simulink library "Autonomous_lib"  (R2023b)
settings: Solver=VariableStepAuto  StartTime=0.0  StopTime=10.0  RelTol=1e-3
undefined symbols (not defined in the file): All_Paths, FloorDistance
libraries: simulink x3
settings Model: Creator=FIRSTMentor  LastModifiedBy=FIRSTMentor

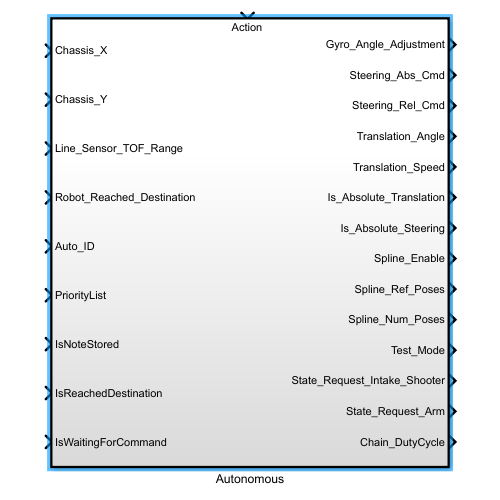
[thumbnail: Simulink's stored preview of the top-level diagram]
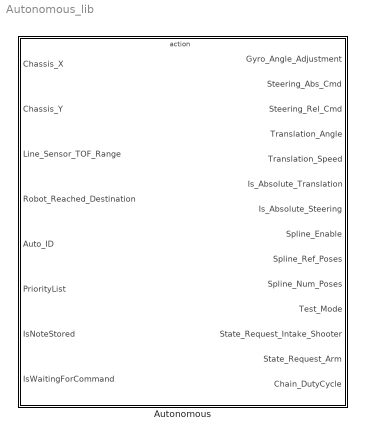
== system Autonomous_lib ==
  Autonomous : Subsystem  TreatAsAtomicUnit=on

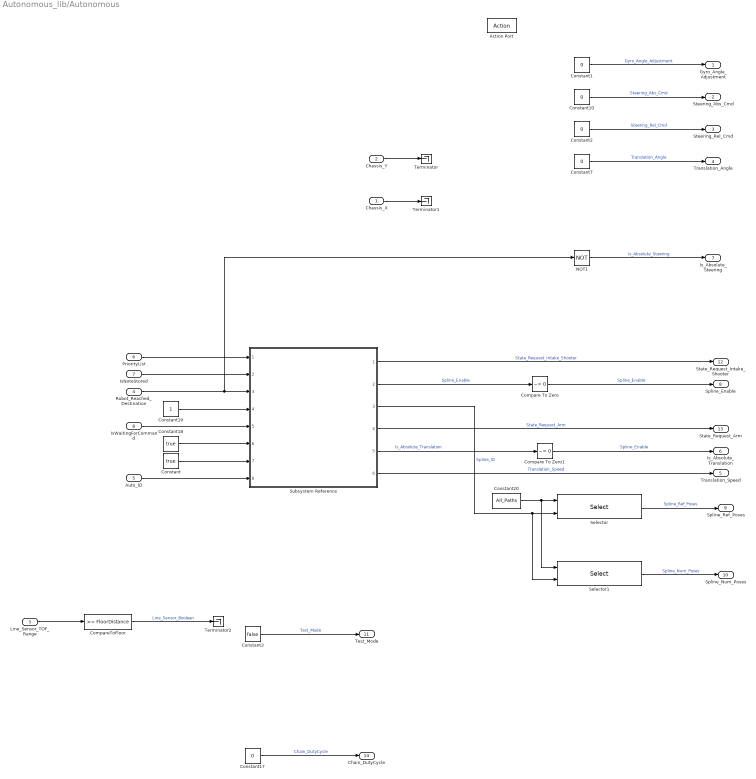
== system Autonomous_lib/Autonomous ==
  Chassis_X : Inport
  Chassis_Y : Inport  Port=2
  Line_Sensor_TOF_Range : Inport  Port=3
  Robot_Reached_Destination : Inport  Port=4
  Auto_ID : Inport  Port=5
  PriorityList : Inport  Port=6
  IsNoteStored : Inport  Port=7
  IsWaitingForCommand : Inport  Port=8
  Action Port : ActionPort  InitializeStates=reset
  Compare To Zero : simulink/Logic and Bit Operations/Compare To Zero  relop=~=  OutDataTypeStr=boolean
  Compare To Zero1 : simulink/Logic and Bit Operations/Compare To Zero  relop=~=  OutDataTypeStr=boolean
  CompareToFloor : simulink/Logic and Bit Operations/Compare To Constant  relop=>=  const=FloorDistance  OutDataTypeStr=boolean
  Constant : Constant  Value=true
  Constant{1..2,7,10,17} (5 alike) : Constant  Value=0
  Constant18 : Constant  Value=true
  Constant19 : Constant
  Constant20 : Constant  Value=All_Paths
  Constant3 : Constant  Value=false  OutDataTypeStr=boolean
  NOT1 : Logic  Operator=NOT  AllPortsSameDT=off  OutDataTypeStr=boolean
  Selector : Selector  NumberOfDimensions=2  InputPortWidth=3  IndexOptions=Index vector (port),Index vector (dialog)  Indices=[1 3],1  OutputSizes=1,1
  Selector1 : Selector  NumberOfDimensions=2  InputPortWidth=3  IndexOptions=Index vector (port),Index vector (dialog)  Indices=[1 3],2  OutputSizes=1,1
  Subsystem Reference : Subsystem  ReferencedSubsystem=State_Interpreter
  Terminator : Terminator
  Terminator1 : Terminator
  Terminator2 : Terminator
  Gyro_Angle_Adjustment : Outport
  Steering_Abs_Cmd : Outport  Port=2
  Steering_Rel_Cmd : Outport  Port=3
  Translation_Angle : Outport  Port=4
  Translation_Speed : Outport  Port=5
  Is_Absolute_Translation : Outport  Port=6
  Is_Absolute_Steering : Outport  Port=7
  Spline_Enable : Outport  Port=8
  Spline_Ref_Poses : Outport  Port=9
  Spline_Num_Poses : Outport  Port=10
  Test_Mode : Outport  Port=11
  State_Request_Intake_Shooter : Outport  Port=12
  State_Request_Arm : Outport  Port=13
  Chain_DutyCycle : Outport  Port=14
  wires:
  Subsystem Reference/5 -> Compare To Zero1/1  "Is_Absolute_Translation"
  Constant2/1 -> Steering_Rel_Cmd/1  "Steering_Rel_Cmd"
  Constant10/1 -> Steering_Abs_Cmd/1  "Steering_Abs_Cmd"
  Constant1/1 -> Gyro_Angle_Adjustment/1  "Gyro_Angle_Adjustment"
  Selector/1 -> Spline_Ref_Poses/1  "Spline_Ref_Poses"
  Selector1/1 -> Spline_Num_Poses/1  "Spline_Num_Poses"
  Chassis_Y/1 -> Terminator/1
  Chassis_X/1 -> Terminator1/1
  Constant7/1 -> Translation_Angle/1  "Translation_Angle"
  Subsystem Reference/6 -> Translation_Speed/1  "Translation_Speed"
  Subsystem Reference/3 -> Selector1/2, Selector/2  "Spline_ID"
  NOT1/1 -> Is_Absolute_Steering/1  "Is_Absolute_Steering"
  Constant3/1 -> Test_Mode/1  "Test_Mode"
  Subsystem Reference/4 -> State_Request_Arm/1  "State_Request_Arm"
  Subsystem Reference/1 -> State_Request_Intake_Shooter/1  "State_Request_Intake_Shooter"
  CompareToFloor/1 -> Terminator2/1  "Line_Sensor_Boolean"
  Line_Sensor_TOF_Range/1 -> CompareToFloor/1
  Constant17/1 -> Chain_DutyCycle/1  "Chain_DutyCycle"
  Auto_ID/1 -> Subsystem Reference/8
  Constant/1 -> Subsystem Reference/7
  PriorityList/1 -> Subsystem Reference/1
  Constant18/1 -> Subsystem Reference/6
  Constant19/1 -> Subsystem Reference/4
  Robot_Reached_Destination/1 -> NOT1/1, Subsystem Reference/3
  IsNoteStored/1 -> Subsystem Reference/2
  IsWaitingForCommand/1 -> Subsystem Reference/5
  Constant20/1 -> Selector1/1, Selector/1
  Subsystem Reference/2 -> Compare To Zero/1  "Spline_Enable"
  Compare To Zero/1 -> Spline_Enable/1  "Spline_Enable"
  Compare To Zero1/1 -> Is_Absolute_Translation/1  "Spline_Enable"
